simulink model "que4"  (R2015a)
settings: Solver=ode45  StartTime=0.0  StopTime=10.0  RelTol=1e-3
libraries: simulink x1
settings Model: Creator=Student  LastModifiedBy=Student

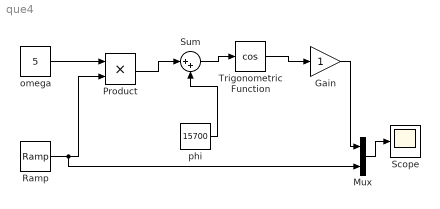
== system que4 ==
  Gain : Gain
  Mux : Mux  Inputs=2
  Product : Product
  Ramp : simulink/Sources/Ramp  slope=1  start=0  X0=0
  Scope : Scope
  Sum : Sum  Inputs=|++
  Trigonometric Function : Trigonometry  Operator=cos
  omega : Constant  Value=5
  phi : Constant  Value=15700
  wires:
  omega/1 -> Product/1
  Ramp/1 -> Mux/2, Product/2
  Gain/1 -> Mux/1
  Mux/1 -> Scope/1
  Product/1 -> Sum/1
  Sum/1 -> Trigonometric Function/1
  Trigonometric Function/1 -> Gain/1
  phi/1 -> Sum/2
